simulink model "Cell_v1"  (R2012b)
settings: Solver=ode45  StartTime=0.0  StopTime=1000  RelTol=1e-3
values from neighbouring files (symbols this model uses):
  l_addasrna_rate_1 = g_addasrna_rate    (= 0)    [run_cell.m]
  l_addasrna_rate_2 = g_addasrna_rate    (= 0)    [run_cell.m]
  l_addasrna_rate_3 = 0.01    [run_cell.m]
  l_addasrna_rate_4 = g_addasrna_rate    (= 0)    [run_cell.m]
  l_asrna_die_rate = 0.01    [run_cell.m]
  l_eaten_rate = 0.001    [run_cell.m]
  l_nuk_die_rate = 0.009    [run_cell.m]
  l_pol_die_rate = 0.01    [run_cell.m]
  l_queue_time = 1    [run_cell.m]
  l_rib_die_rate = 0.004    [run_cell.m]
  l_rib_serv_rate = 0.01    [run_cell.m]
  n_asrna = 3    [run_cell.m]
  n_rib = n_initial_rib    (= 15)    [run_cell.m]
  n_rnk_nuk = a    (= 15)    [run_cell.m]
  n_rnk_pol = n_initial_pol    (= 15)    [run_cell.m]
  seed = (seed-321)    (= 12025)    [run_cell.m]
undefined symbols (not defined in the file or in its folder): des, gcbh, PacketRate
libraries: simulink x3
settings Model: Creator=Alex  LastModifiedBy=Alex
settings DataIOCC: InspectSignalLogs=on
settings ConfigurationSet: Description=SimMechanics 2G

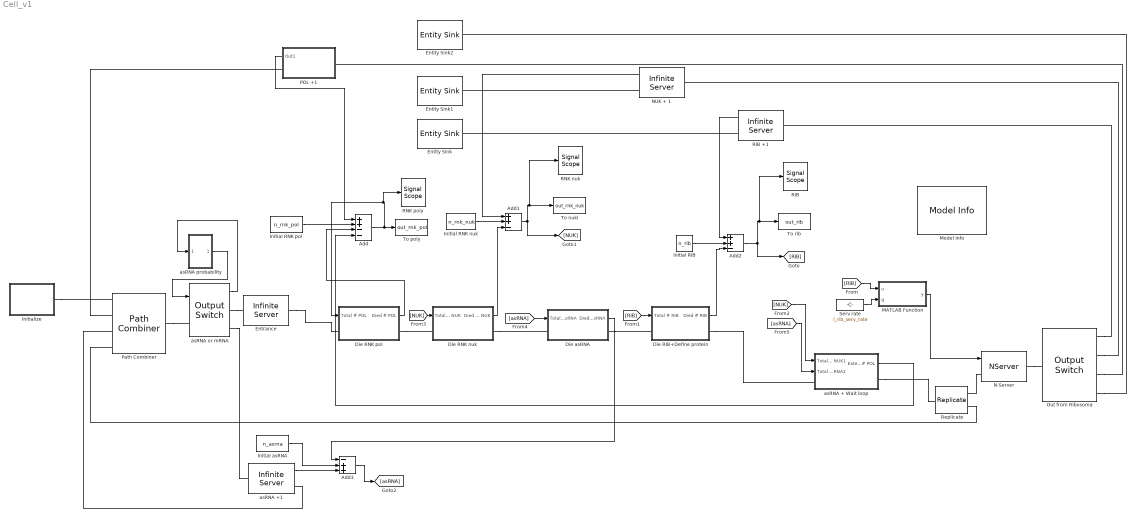
== system Cell_v1 ==
  Add : Sum  Inputs=++--
  Add1 : Sum  Inputs=++-
  Add2 : Sum  Inputs=++-
  Add3 : Sum  Inputs=-++
  Die RIB+Define protein : Subsystem
  Die RNK nuk : Subsystem
  Die RNK pol : Subsystem
  Die asRNA : Subsystem
  Entity Sink : EntitySink
  Entity Sink1 : EntitySink
  Entity Sink2 : EntitySink
  Entrance : InfiniteServer  ServiceTime=0
  Initial RIB : Constant  Value=n_rib
  Initial RNK nuk : Constant  Value=n_rnk_nuk
  Initial RNK pol : Constant  Value=n_rnk_pol
  Initial asRNA : Constant  Value=n_asrna
  Initialize : Subsystem
  MATLAB Function : MATLAB Function  TreatAsAtomicUnit=on
  Model Info : simulink/Model-Wide Utilities/Model Info  InitialBlockCM=None  BlockCM=None  Frame=on  DisplayStringWithTags=|  HorizontalTextAlignment=Center  LeftAlignmentValue=0.5  SourceBlockDiagram=Cell_v1  TagMaxNumber=20
      | Model Info
      | 1 - Ribosome
      | 2 - RNK nuclease
      | 3 - RNK polymerase
  N-Server : NServer  NumberOfServers=n_rib  ServiceTimeFrom=Signal port t  ServiceTime=2
  NUK + 1 : InfiniteServer  ServiceTime=0  StatNumberDeparted=on
  Out from Ribosoma : OutputSwitch  NumberOutputPorts=4  SwitchingCriterion=From attribute  AttributeName=Protein
  POL +1 : Subsystem
  Path Combiner : PathCombiner  NumberInputPorts=4
  RIB : SignalScope  LoadFcn=des.scope.CallbackSupport('seLoadFcn',gcbh)  StartFcn=des.scope.CallbackSupport('seStartFcn',gcbh)  StopFcn=des.scope.CallbackSupport('seStopFcn',gcbh)  XLabel=Time  YLabel=Total Number of Entities  ShowCountPlotted=on  DataStoreOption=Unlimited
      settings: CopyFcn=des.scope.CallbackSupport('seCopyFcn',gcbh)  DeleteFcn=des.scope.CallbackSupport('seDeleteFcn',gcbh)  PreSaveFcn=des.scope.CallbackSupport('sePreSaveFcn',gcbh)  NameChangeFcn=des.scope.CallbackSupport('seNameChangeFcn',gcbh)  OpenFcn=des.scope.CallbackSupport('seOpenFcn',gcbh)
  RIB +1 : InfiniteServer  ServiceTime=0  StatNumberDeparted=on
  RNK nuk : SignalScope  LoadFcn=des.scope.CallbackSupport('seLoadFcn',gcbh)  StartFcn=des.scope.CallbackSupport('seStartFcn',gcbh)  StopFcn=des.scope.CallbackSupport('seStopFcn',gcbh)  XLabel=Time  YLabel=Total Number of Entities  DataStoreOption=Unlimited
      settings: CopyFcn=des.scope.CallbackSupport('seCopyFcn',gcbh)  DeleteFcn=des.scope.CallbackSupport('seDeleteFcn',gcbh)  PreSaveFcn=des.scope.CallbackSupport('sePreSaveFcn',gcbh)  NameChangeFcn=des.scope.CallbackSupport('seNameChangeFcn',gcbh)  OpenFcn=des.scope.CallbackSupport('seOpenFcn',gcbh)
  RNK poly : SignalScope  LoadFcn=des.scope.CallbackSupport('seLoadFcn',gcbh)  StartFcn=des.scope.CallbackSupport('seStartFcn',gcbh)  StopFcn=des.scope.CallbackSupport('seStopFcn',gcbh)  XLabel=Time  YLabel=Total Number of Entities  DataStoreOption=Unlimited
      settings: CopyFcn=des.scope.CallbackSupport('seCopyFcn',gcbh)  DeleteFcn=des.scope.CallbackSupport('seDeleteFcn',gcbh)  PreSaveFcn=des.scope.CallbackSupport('sePreSaveFcn',gcbh)  NameChangeFcn=des.scope.CallbackSupport('seNameChangeFcn',gcbh)  OpenFcn=des.scope.CallbackSupport('seOpenFcn',gcbh)
  Replicate : Replicate  NumberOutputPorts=2
  Serv rate : Constant  Value=l_rib_serv_rate
  To nukl : ToWorkspace  VariableName=out_rnk_nuk  SampleTime=-1  SaveFormat=Timeseries
  To poly : ToWorkspace  VariableName=out_rnk_pol  SampleTime=-1  SaveFormat=Timeseries
  To rib : ToWorkspace  VariableName=out_rib  SampleTime=-1  SaveFormat=Timeseries
  asRNA + Wait loop : Subsystem
  asRNA +1 : InfiniteServer  ServiceTime=0  StatNumberDeparted=on
  asRNA or mRNA : OutputSwitch  NumberOutputPorts=2  SwitchingCriterion=From signal port p  StatNumberDeparted=on
  asRNA probability : Subsystem
  wires:
  Die RNK nuk/1(Died # NUK) -> Add1/3
  Die RIB+Define protein/1(Died # RIB) -> Add2/3
  Die RNK pol/1(Died # POL) -> Add/3
  NUK + 1/1 -> Add1/1
  Add1/1 -> RNK nuk/1, To nukl/1, [NUK]
  RIB +1/1 -> Add2/1
  Add/1 -> To poly/1, RNK poly/1, Die RNK pol/1(Total # POL)
  Initial RNK pol/1 -> Add/2
  Initial RNK nuk/1 -> Add1/2
  Initial RIB/1 -> Add2/2
  MATLAB Function/1(y) -> N-Server/1
  POL +1/1(Out1) -> Add/1
  asRNA + Wait loop/1(Eaten # POL) -> Add/4
  [RIB] -> MATLAB Function/1(u)
  [RIB] -> Die RIB+Define protein/1(Total # RIB)
  Add2/1 -> RIB/1, To rib/1, [RIB]
  [NUK] -> asRNA + Wait loop/1(Total # NUK1)
  [NUK] -> Die RNK nuk/1(Total # NUK)
  Serv rate/1 -> MATLAB Function/2(g)
  asRNA or mRNA/1 -> asRNA probability/1(In1)
  asRNA probability/1(Out1) -> asRNA or mRNA/1
  asRNA +1/1 -> Add3/3
  Initial asRNA/1 -> Add3/2
  [asRNA] -> Die asRNA/1(Total # asRNA)
  Die asRNA/1(Died # asRNA) -> Add3/1
  [asRNA] -> asRNA + Wait loop/2(Total # asRNA2)
  Add3/1 -> [asRNA]
  connections:
  RIB +1/RConn1 -- Entity Sink/LConn1
  Out from Ribosoma/RConn2 -- NUK + 1/LConn1
  NUK + 1/RConn1 -- Entity Sink1/LConn1
  Out from Ribosoma/RConn1 -- RIB +1/LConn1
  Initialize/RConn1 -- Path Combiner/LConn1
  Die RNK pol/RConn1 -- Die RNK nuk/LConn1
  Die asRNA/RConn1 -- Die RIB+Define protein/LConn1
  Entrance/RConn1 -- Die RNK pol/LConn1
  Out from Ribosoma/RConn4 -- Entity Sink2/LConn1
  POL +1/RConn1 -- Path Combiner/LConn2
  Out from Ribosoma/RConn3 -- POL +1/LConn1
  asRNA + Wait loop/RConn1 -- Replicate/LConn1
  N-Server/RConn1 -- Out from Ribosoma/LConn1
  Replicate/RConn1 -- N-Server/LConn1
  Replicate/RConn2 -- Path Combiner/LConn4
  Path Combiner/RConn1 -- asRNA or mRNA/LConn1
  asRNA or mRNA/RConn1 -- Entrance/LConn1
  asRNA or mRNA/RConn2 -- asRNA +1/LConn1
  asRNA +1/RConn1 -- Path Combiner/LConn3
  Die RNK nuk/RConn1 -- Die asRNA/LConn1
  Die RIB+Define protein/RConn1 -- asRNA + Wait loop/LConn1

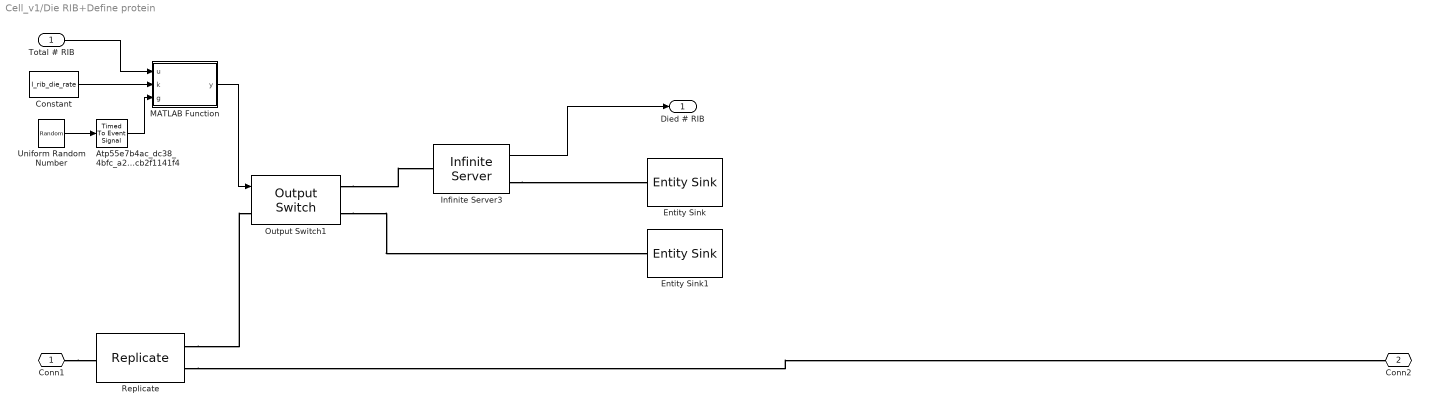
== system Cell_v1/Die RIB+Define protein ==
  Total # RIB : Inport
  Atp55e7b4ac_dc38_4bfc_a2da_90cb2f1141f4 : TimedToEventSignal
  Constant : Constant  Value=l_rib_die_rate
  Entity Sink : EntitySink
  Entity Sink1 : EntitySink
  Infinite Server3 : InfiniteServer  ServiceTime=0  StatNumberDeparted=on
  MATLAB Function : MATLAB Function  TreatAsAtomicUnit=on
  Output Switch1 : OutputSwitch  NumberOutputPorts=2  SwitchingCriterion=From signal port p  InitialConditionsOpt=on  InitialConditions=2
  Replicate : Replicate  NumberOutputPorts=2
  Uniform Random Number : UniformRandomNumber  Minimum=-0.5  Maximum=0.5  Seed=seed  SampleTime=0
  Conn1 : PMIOPort  Port=1  Side=Left
  Conn2 : PMIOPort  Port=2  Side=Right
  Died # RIB : Outport
  wires:
  Infinite Server3/1 -> Died # RIB/1
  MATLAB Function/1(y) -> Output Switch1/1
  Uniform Random Number/1 -> Atp55e7b4ac_dc38_4bfc_a2da_90cb2f1141f4/1
  Atp55e7b4ac_dc38_4bfc_a2da_90cb2f1141f4/1 -> MATLAB Function/3(g)
  Total # RIB/1 -> MATLAB Function/1(u)
  Constant/1 -> MATLAB Function/2(k)
  connections:
  Replicate/RConn1 -- Output Switch1/LConn1
  Infinite Server3/RConn1 -- Entity Sink/LConn1
  Conn1/RConn1 -- Replicate/LConn1
  Output Switch1/RConn1 -- Infinite Server3/LConn1
  Output Switch1/RConn2 -- Entity Sink1/LConn1
  Replicate/RConn2 -- Conn2/RConn1

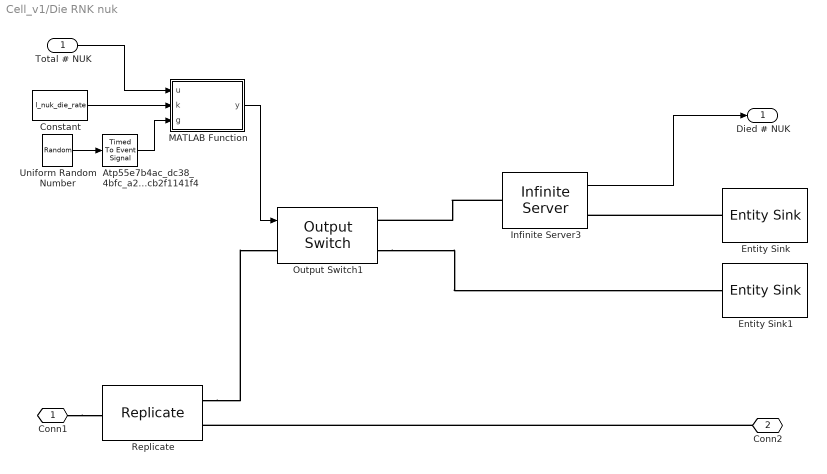
== system Cell_v1/Die RNK nuk ==
  Total # NUK : Inport
  Atp55e7b4ac_dc38_4bfc_a2da_90cb2f1141f4 : TimedToEventSignal
  Constant : Constant  Value=l_nuk_die_rate
  Entity Sink : EntitySink
  Entity Sink1 : EntitySink
  Infinite Server3 : InfiniteServer  ServiceTime=0  StatNumberDeparted=on
  MATLAB Function : MATLAB Function  TreatAsAtomicUnit=on
  Output Switch1 : OutputSwitch  NumberOutputPorts=2  SwitchingCriterion=From signal port p  InitialConditionsOpt=on  InitialConditions=2
  Replicate : Replicate  NumberOutputPorts=2
  Uniform Random Number : UniformRandomNumber  Minimum=-0.5  Maximum=0.5  Seed=seed  SampleTime=0
  Conn1 : PMIOPort  Port=1  Side=Left
  Conn2 : PMIOPort  Port=2  Side=Right
  Died # NUK : Outport
  wires:
  Infinite Server3/1 -> Died # NUK/1
  MATLAB Function/1(y) -> Output Switch1/1
  Uniform Random Number/1 -> Atp55e7b4ac_dc38_4bfc_a2da_90cb2f1141f4/1
  Atp55e7b4ac_dc38_4bfc_a2da_90cb2f1141f4/1 -> MATLAB Function/3(g)
  Total # NUK/1 -> MATLAB Function/1(u)
  Constant/1 -> MATLAB Function/2(k)
  connections:
  Entity Sink/LConn1 -- Infinite Server3/RConn1
  Replicate/RConn1 -- Output Switch1/LConn1
  Conn1/RConn1 -- Replicate/LConn1
  Conn2/RConn1 -- Replicate/RConn2
  Infinite Server3/LConn1 -- Output Switch1/RConn1
  Output Switch1/RConn2 -- Entity Sink1/LConn1

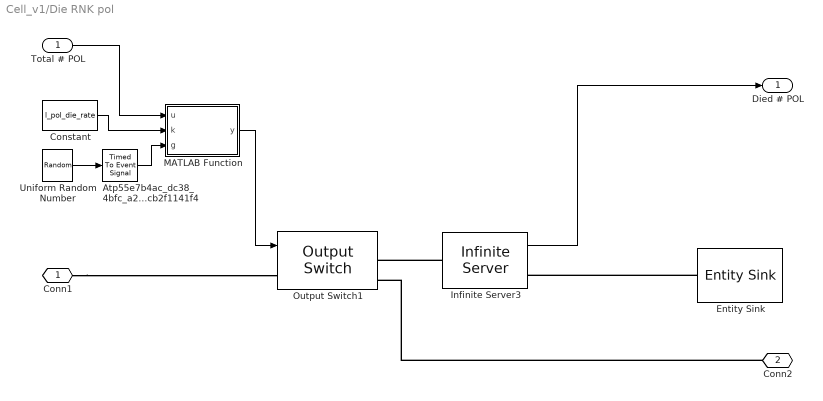
== system Cell_v1/Die RNK pol ==
  Total # POL : Inport
  Atp55e7b4ac_dc38_4bfc_a2da_90cb2f1141f4 : TimedToEventSignal
  Constant : Constant  Value=l_pol_die_rate
  Entity Sink : EntitySink
  Infinite Server3 : InfiniteServer  ServiceTime=0  StatNumberDeparted=on
  MATLAB Function : MATLAB Function  TreatAsAtomicUnit=on
  Output Switch1 : OutputSwitch  NumberOutputPorts=2  SwitchingCriterion=From signal port p  InitialConditionsOpt=on  InitialConditions=2  StatLastDeparturePort=on
      settings: OutputPortMap=o3
  Uniform Random Number : UniformRandomNumber  Minimum=-0.5  Maximum=0.5  Seed=seed  SampleTime=0
  Conn1 : PMIOPort  Port=1  Side=Left
  Conn2 : PMIOPort  Port=2  Side=Right
  Died # POL : Outport
  wires:
  Infinite Server3/1 -> Died # POL/1
  Uniform Random Number/1 -> Atp55e7b4ac_dc38_4bfc_a2da_90cb2f1141f4/1
  Atp55e7b4ac_dc38_4bfc_a2da_90cb2f1141f4/1 -> MATLAB Function/3(g)
  Total # POL/1 -> MATLAB Function/1(u)
  MATLAB Function/1(y) -> Output Switch1/1
  Constant/1 -> MATLAB Function/2(k)
  connections:
  Entity Sink/LConn1 -- Infinite Server3/RConn1
  Infinite Server3/LConn1 -- Output Switch1/RConn1
  Conn2/RConn1 -- Output Switch1/RConn2
  Conn1/RConn1 -- Output Switch1/LConn1

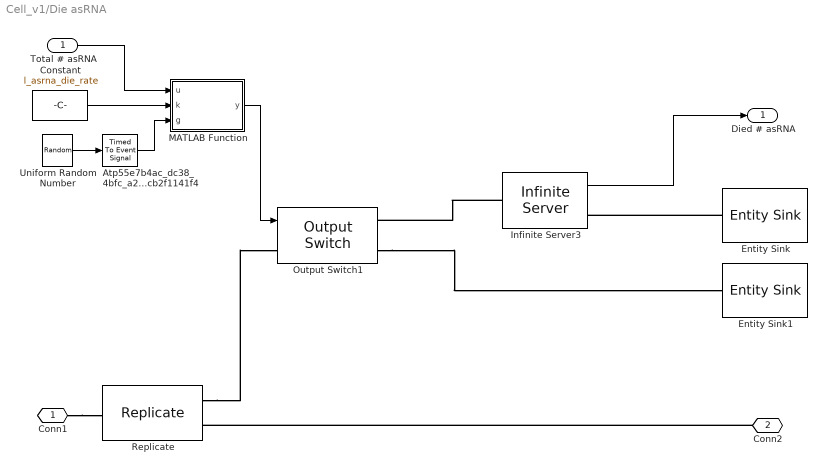
== system Cell_v1/Die asRNA ==
  Total # asRNA : Inport
  Atp55e7b4ac_dc38_4bfc_a2da_90cb2f1141f4 : TimedToEventSignal
  Constant : Constant  Value=l_asrna_die_rate
  Entity Sink : EntitySink
  Entity Sink1 : EntitySink
  Infinite Server3 : InfiniteServer  ServiceTime=0  StatNumberDeparted=on
  MATLAB Function : MATLAB Function  TreatAsAtomicUnit=on
  Output Switch1 : OutputSwitch  NumberOutputPorts=2  SwitchingCriterion=From signal port p  InitialConditionsOpt=on  InitialConditions=2
  Replicate : Replicate  NumberOutputPorts=2
  Uniform Random Number : UniformRandomNumber  Minimum=-0.5  Maximum=0.5  Seed=seed  SampleTime=0
  Conn1 : PMIOPort  Port=1  Side=Left
  Conn2 : PMIOPort  Port=2  Side=Right
  Died # asRNA : Outport
  wires:
  Infinite Server3/1 -> Died # asRNA/1
  MATLAB Function/1(y) -> Output Switch1/1
  Uniform Random Number/1 -> Atp55e7b4ac_dc38_4bfc_a2da_90cb2f1141f4/1
  Atp55e7b4ac_dc38_4bfc_a2da_90cb2f1141f4/1 -> MATLAB Function/3(g)
  Total # asRNA/1 -> MATLAB Function/1(u)
  Constant/1 -> MATLAB Function/2(k)
  connections:
  Entity Sink/LConn1 -- Infinite Server3/RConn1
  Replicate/RConn1 -- Output Switch1/LConn1
  Conn1/RConn1 -- Replicate/LConn1
  Conn2/RConn1 -- Replicate/RConn2
  Infinite Server3/LConn1 -- Output Switch1/RConn1
  Output Switch1/RConn2 -- Entity Sink1/LConn1

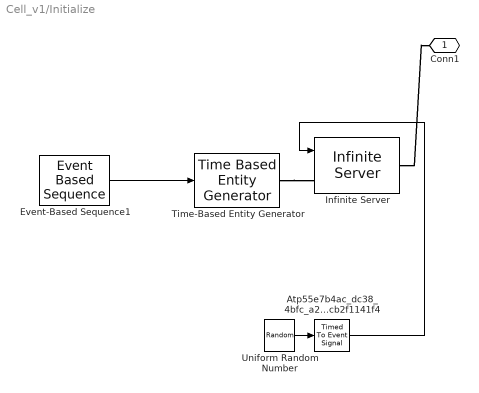
== system Cell_v1/Initialize ==
  Atp55e7b4ac_dc38_4bfc_a2da_90cb2f1141f4 : TimedToEventSignal
  Event-Based Sequence1 : EventBasedSequence  VectorOutputValues=p_initial_pol  FormOutputOpt=Setting to infinity
  Infinite Server : InfiniteServer  ServiceTimeFrom=Signal port t
  Time-Based Entity Generator : TimeBasedEntityGenerator  GenerateEntitiesUpon=Intergeneration time from port t  Distribution=Uniform
  Uniform Random Number : UniformRandomNumber  Minimum=0  Seed=seed  SampleTime=0
  Conn1 : PMIOPort  Port=1  Side=Right
  wires:
  Uniform Random Number/1 -> Atp55e7b4ac_dc38_4bfc_a2da_90cb2f1141f4/1
  Event-Based Sequence1/1 -> Time-Based Entity Generator/1
  Atp55e7b4ac_dc38_4bfc_a2da_90cb2f1141f4/1 -> Infinite Server/1
  connections:
  Time-Based Entity Generator/RConn1 -- Infinite Server/LConn1
  Infinite Server/RConn1 -- Conn1/RConn1

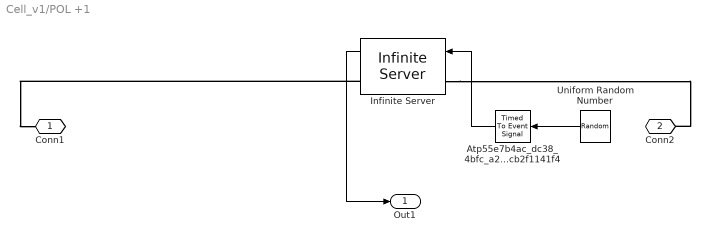
== system Cell_v1/POL +1 ==
  Atp55e7b4ac_dc38_4bfc_a2da_90cb2f1141f4 : TimedToEventSignal
  Infinite Server : InfiniteServer  ServiceTimeFrom=Signal port t  ServiceTime=0  StatNumberDeparted=on
  Uniform Random Number : UniformRandomNumber  Minimum=0  Seed=seed  SampleTime=0
  Conn1 : PMIOPort  Port=1  Side=Right
  Conn2 : PMIOPort  Port=2  Side=Left
  Out1 : Outport
  wires:
  Infinite Server/1 -> Out1/1
  Uniform Random Number/1 -> Atp55e7b4ac_dc38_4bfc_a2da_90cb2f1141f4/1
  Atp55e7b4ac_dc38_4bfc_a2da_90cb2f1141f4/1 -> Infinite Server/1
  connections:
  Infinite Server/LConn1 -- Conn2/RConn1
  Infinite Server/RConn1 -- Conn1/RConn1

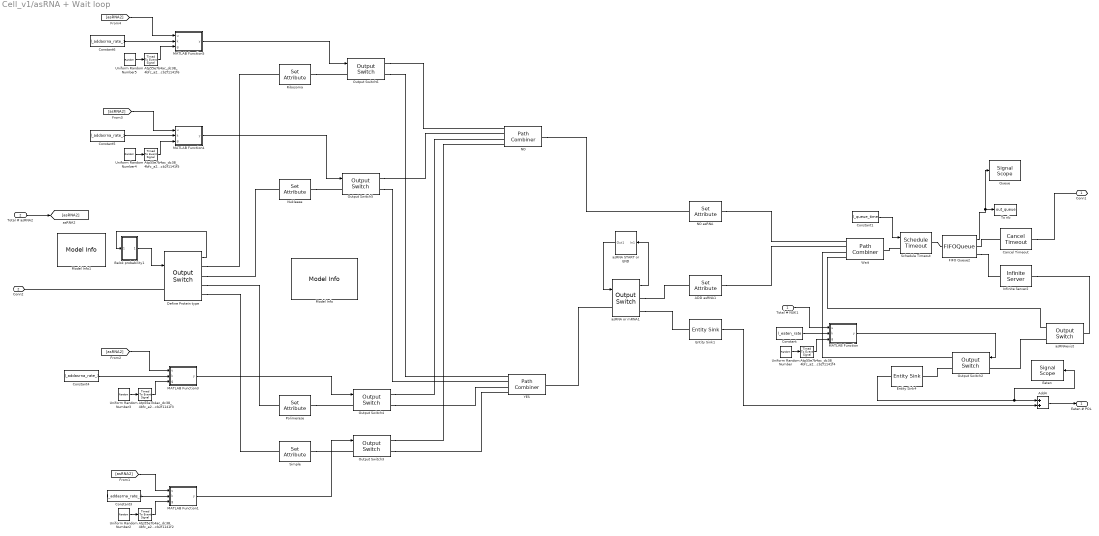
== system Cell_v1/asRNA + Wait loop ==
  Total # NUK1 : Inport
  Total # asRNA2 : Inport  Port=2
  ADD asRNA1 : SetAttribute  AttributeName=asRNAexist  EvaluatedAttributeValue={ 1 }
  Add4 : Sum
  Atp55e7b4ac_dc38_4bfc_a2da_90cb2f1141f{2..6} (5 alike) : TimedToEventSignal
  Belok probability1 : Subsystem
  Cancel Timeout : CancelTimeout
  Constant : Constant  Value=l_eaten_rate
  Constant1 : Constant  Value=l_queue_time
  Constant3 : Constant  Value=l_addasrna_rate_4
  Constant4 : Constant  Value=l_addasrna_rate_3
  Constant5 : Constant  Value=l_addasrna_rate_2
  Constant6 : Constant  Value=l_addasrna_rate_1
  Define Protein type : OutputSwitch  NumberOutputPorts=4  SwitchingCriterion=From signal port p  StatNumberDeparted=on
  Eaten : SignalScope  LoadFcn=des.scope.CallbackSupport('seLoadFcn',gcbh)  StartFcn=des.scope.CallbackSupport('seStartFcn',gcbh)  StopFcn=des.scope.CallbackSupport('seStopFcn',gcbh)
      settings: CopyFcn=des.scope.CallbackSupport('seCopyFcn',gcbh)  DeleteFcn=des.scope.CallbackSupport('seDeleteFcn',gcbh)  PreSaveFcn=des.scope.CallbackSupport('sePreSaveFcn',gcbh)  NameChangeFcn=des.scope.CallbackSupport('seNameChangeFcn',gcbh)  OpenFcn=des.scope.CallbackSupport('seOpenFcn',gcbh)
  Entity Sink1 : EntitySink  StatNumberArrived=on
  Entity Sink4 : EntitySink  StatNumberArrived=on
  FIFO Queue2 : FIFOQueue  Capacity=10000  EnableTOPort=on  StatAverageQueueLength=on
      settings: OutputPortMap=o3
  Infinite Server2 : InfiniteServer  ServiceTime=0
  MATLAB Function : MATLAB Function  TreatAsAtomicUnit=on
  MATLAB Function1 : MATLAB Function  TreatAsAtomicUnit=on
  MATLAB Function3 : MATLAB Function  TreatAsAtomicUnit=on
  MATLAB Function4 : MATLAB Function  TreatAsAtomicUnit=on
  MATLAB Function5 : MATLAB Function  TreatAsAtomicUnit=on
  Model Info : simulink/Model-Wide Utilities/Model Info  InitialBlockCM=None  BlockCM=None  Frame=on  DisplayStringWithTags=|  HorizontalTextAlignment=Center  LeftAlignmentValue=0.5  SourceBlockDiagram=Cell_v1  TagMaxNumber=20
      | Add asRNA
      | 1 - NO, asRNA was NOT added
      | 2 - YES, asRNA was added
  Model Info1 : simulink/Model-Wide Utilities/Model Info  InitialBlockCM=None  BlockCM=None  Frame=on  DisplayStringWithTags=|  HorizontalTextAlignment=Center  LeftAlignmentValue=0.5  SourceBlockDiagram=Cell_v1  TagMaxNumber=20
      | Model Info
      | 1 - Ribosome
      | 2 - RNK nuclease
      | 3 - RNK polymerase
  NO : PathCombiner  NumberInputPorts=4
  NO asRNA : SetAttribute  AttributeName=asRNAexist  AttributeValue=2  EvaluatedAttributeValue={ 2 }
  Nuklease : SetAttribute  AttributeName=Protein  AttributeValue=2  EvaluatedAttributeValue={ 2 }
  Output Switch2 : OutputSwitch  NumberOutputPorts=2  SwitchingCriterion=From signal port p  InitialConditionsOpt=on
  Output Switch{3..6} (4 alike) : OutputSwitch  NumberOutputPorts=2  SwitchingCriterion=From signal port p
  Polimerase : SetAttribute  AttributeName=Protein  AttributeValue=3  EvaluatedAttributeValue={ 3 }
  Queue : SignalScope  LoadFcn=des.scope.CallbackSupport('seLoadFcn',gcbh)  StartFcn=des.scope.CallbackSupport('seStartFcn',gcbh)  StopFcn=des.scope.CallbackSupport('seStopFcn',gcbh)
      settings: CopyFcn=des.scope.CallbackSupport('seCopyFcn',gcbh)  DeleteFcn=des.scope.CallbackSupport('seDeleteFcn',gcbh)  PreSaveFcn=des.scope.CallbackSupport('sePreSaveFcn',gcbh)  NameChangeFcn=des.scope.CallbackSupport('seNameChangeFcn',gcbh)  OpenFcn=des.scope.CallbackSupport('seOpenFcn',gcbh)
  Ribosoma : SetAttribute  AttributeName=Protein  EvaluatedAttributeValue={ 1 }
  Schedule Timeout : ScheduleTimeout  TimeoutIntervalFrom=Signal port ti  TimeoutInterval=2
  Simple : SetAttribute  AttributeName=Protein  AttributeValue=4  EvaluatedAttributeValue={ 4 }
  To rib : ToWorkspace  VariableName=out_queue  SampleTime=-1  SaveFormat=Timeseries
  Uniform Random Number{,2..5} (5 alike) : UniformRandomNumber  Minimum=-0.5  Maximum=0.5  Seed=seed  SampleTime=0
  Wait : PathCombiner  NumberInputPorts=4
  YES : PathCombiner  NumberInputPorts=4
  asRNA START or END : Subsystem
  asRNA or mRNA1 : OutputSwitch  NumberOutputPorts=2  SwitchingCriterion=From signal port p  StatNumberDeparted=on
  asRNAexist : OutputSwitch  NumberOutputPorts=2  SwitchingCriterion=From attribute  AttributeName=asRNAexist  InitialConditionsOpt=on
  Conn1 : PMIOPort  Port=1  Side=Right
  Conn2 : PMIOPort  Port=2  Side=Left
  Eaten # POL : Outport
  wires:
  Entity Sink4/1 -> Eaten/1, Add4/1
  Uniform Random Number/1 -> Atp55e7b4ac_dc38_4bfc_a2da_90cb2f1141f4/1
  Atp55e7b4ac_dc38_4bfc_a2da_90cb2f1141f4/1 -> MATLAB Function/3(g)
  Total # NUK1/1 -> MATLAB Function/1(u)
  MATLAB Function/1(y) -> Output Switch2/1
  Constant/1 -> MATLAB Function/2(k)
  Constant1/1 -> Schedule Timeout/1
  asRNA or mRNA1/1 -> asRNA START or END/1(In1)
  asRNA START or END/1(Out1) -> asRNA or mRNA1/1
  Entity Sink1/1 -> Add4/2
  Add4/1 -> Eaten # POL/1
  Define Protein type/1 -> Belok probability1/1(In1)
  Belok probability1/1(Out1) -> Define Protein type/1
  Uniform Random Number2/1 -> Atp55e7b4ac_dc38_4bfc_a2da_90cb2f1141f2/1
  Atp55e7b4ac_dc38_4bfc_a2da_90cb2f1141f2/1 -> MATLAB Function1/3(g)
  Constant3/1 -> MATLAB Function1/2(k)
  MATLAB Function1/1(y) -> Output Switch3/1
  Uniform Random Number3/1 -> Atp55e7b4ac_dc38_4bfc_a2da_90cb2f1141f3/1
  Atp55e7b4ac_dc38_4bfc_a2da_90cb2f1141f3/1 -> MATLAB Function3/3(g)
  Constant4/1 -> MATLAB Function3/2(k)
  MATLAB Function3/1(y) -> Output Switch4/1
  Uniform Random Number4/1 -> Atp55e7b4ac_dc38_4bfc_a2da_90cb2f1141f5/1
  Atp55e7b4ac_dc38_4bfc_a2da_90cb2f1141f5/1 -> MATLAB Function4/3(g)
  [asRNA2] -> MATLAB Function4/1(u)
  Constant5/1 -> MATLAB Function4/2(k)
  MATLAB Function4/1(y) -> Output Switch5/1
  Uniform Random Number5/1 -> Atp55e7b4ac_dc38_4bfc_a2da_90cb2f1141f6/1
  Atp55e7b4ac_dc38_4bfc_a2da_90cb2f1141f6/1 -> MATLAB Function5/3(g)
  [asRNA2] -> MATLAB Function5/1(u)
  Constant6/1 -> MATLAB Function5/2(k)
  MATLAB Function5/1(y) -> Output Switch6/1
  Total # asRNA2/1 -> [asRNA2]
  [asRNA2] -> MATLAB Function3/1(u)
  [asRNA2] -> MATLAB Function1/1(u)
  FIFO Queue2/1 -> Queue/1, To rib/1
  connections:
  FIFO Queue2/RConn2 -- Infinite Server2/LConn1
  Wait/LConn3 -- Output Switch2/RConn1
  Wait/RConn1 -- Schedule Timeout/LConn1
  Output Switch2/RConn2 -- Entity Sink4/LConn1
  Cancel Timeout/RConn1 -- Conn1/RConn1
  Schedule Timeout/RConn1 -- FIFO Queue2/LConn1
  FIFO Queue2/RConn1 -- Cancel Timeout/LConn1
  Infinite Server2/RConn1 -- asRNAexist/LConn1
  asRNAexist/RConn1 -- Wait/LConn4
  asRNAexist/RConn2 -- Output Switch2/LConn1
  asRNA or mRNA1/LConn1 -- YES/RConn1
  asRNA or mRNA1/RConn1 -- ADD asRNA1/LConn1
  asRNA or mRNA1/RConn2 -- Entity Sink1/LConn1
  NO/RConn1 -- NO asRNA/LConn1
  NO asRNA/RConn1 -- Wait/LConn1
  ADD asRNA1/RConn1 -- Wait/LConn2
  Define Protein type/RConn2 -- Nuklease/LConn1
  Define Protein type/LConn1 -- Conn2/RConn1
  Ribosoma/RConn1 -- Output Switch6/LConn1
  Nuklease/RConn1 -- Output Switch5/LConn1
  Simple/RConn1 -- Output Switch3/LConn1
  Define Protein type/RConn3 -- Polimerase/LConn1
  Define Protein type/RConn1 -- Ribosoma/LConn1
  Define Protein type/RConn4 -- Simple/LConn1
  Polimerase/RConn1 -- Output Switch4/LConn1
  Output Switch6/RConn1 -- NO/LConn1
  Output Switch5/RConn1 -- NO/LConn2
  Output Switch4/RConn1 -- NO/LConn3
  Output Switch3/RConn1 -- NO/LConn4
  Output Switch4/RConn2 -- YES/LConn3
  Output Switch3/RConn2 -- YES/LConn4
  Output Switch6/RConn2 -- YES/LConn1
  Output Switch5/RConn2 -- YES/LConn2

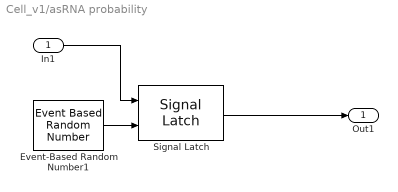
== system Cell_v1/asRNA probability ==
  In1 : Inport
  Event-Based Random Number1 : EventBasedRandomNumber  Distribution=Arbitrary discrete  meanExp=1/PacketRate  minUnif=1  maxUnif=MaxPacketSize  valueVecDisc=[1 2]  probVecDisc=p_RNA_routing  Seed=seed
  Signal Latch : SignalLatch  InitialMemoryValue=2  ReadMemoryUpon=Write to memory event
      settings: InputPortMap=u0,u2  OutputPortMap=o2
  Out1 : Outport
  wires:
  Event-Based Random Number1/1 -> Signal Latch/2
  Signal Latch/1 -> Out1/1
  In1/1 -> Signal Latch/1

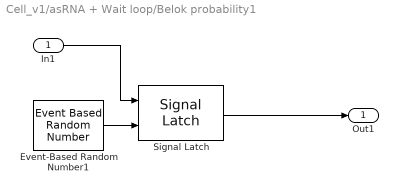
== system Cell_v1/asRNA + Wait loop/Belok probability1 ==
  In1 : Inport
  Event-Based Random Number1 : EventBasedRandomNumber  Distribution=Arbitrary discrete  meanExp=1/PacketRate  minUnif=1  maxUnif=MaxPacketSize  valueVecDisc=[1 2 3 4]  probVecDisc=p_routing  Seed=seed
  Signal Latch : SignalLatch  InitialMemoryValue=2  ReadMemoryUpon=Write to memory event
      settings: InputPortMap=u0,u2  OutputPortMap=o2
  Out1 : Outport
  wires:
  Event-Based Random Number1/1 -> Signal Latch/2
  Signal Latch/1 -> Out1/1
  In1/1 -> Signal Latch/1

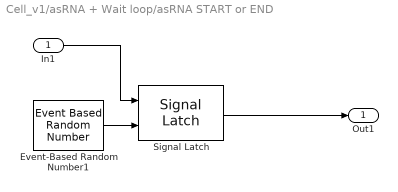
== system Cell_v1/asRNA + Wait loop/asRNA START or END ==
  In1 : Inport
  Event-Based Random Number1 : EventBasedRandomNumber  Distribution=Arbitrary discrete  meanExp=1/PacketRate  minUnif=1  maxUnif=MaxPacketSize  valueVecDisc=[1 2]  probVecDisc=p_asRNA_start_end  Seed=seed
  Signal Latch : SignalLatch  InitialMemoryValue=2  ReadMemoryUpon=Write to memory event
      settings: InputPortMap=u0,u2  OutputPortMap=o2
  Out1 : Outport
  wires:
  Event-Based Random Number1/1 -> Signal Latch/2
  Signal Latch/1 -> Out1/1
  In1/1 -> Signal Latch/1

== matlab function Cell_v1/Die RIB+Define protein/MATLAB Function ==
  data: u input; k input; y output; g input
function y = fcnRIB(u,k,g)
y =1+round(g + exp(-k*u));

== matlab function Cell_v1/MATLAB Function ==
  data: u input; y output; g input
function y = TimeInServer(u,g)
%#codegen
k = rand(1);

y = 10*exp(-g*u)*(1+0.2*(k-0.5));

== matlab function Cell_v1/Die RNK nuk/MATLAB Function ==
  data: u input; k input; y output; g input
function y = fcnNUK(u,k,g)
y =1+round(g + exp(-k*u));

== matlab function Cell_v1/asRNA + Wait loop/MATLAB Function ==
  data: u input; k input; y output; g input
function y = fcnPOL(u,k,g)
y =1+round(g + 1-exp(-k*u));

== matlab function Cell_v1/Die asRNA/MATLAB Function ==
  data: u input; k input; y output; g input
function y = fcnNUK(u,k,g)
y =1+round(g + exp(-k*u));

== matlab function Cell_v1/Die RNK pol/MATLAB Function ==
  data: u input; k input; y output; g input
function y = fcnPOL(u,k,g)
y =1+min(round(g + exp(-k*u)+0.1),1) ;

== matlab function Cell_v1/asRNA + Wait loop/MATLAB Function1 ==
  data: u input; k input; y output; g input
function y = fcnPOL(u,k,g)
y =1+round(g + 1-exp(-k*u));

== matlab function Cell_v1/asRNA + Wait loop/MATLAB Function3 ==
  data: u input; k input; y output; g input
function y = fcnPOL(u,k,g)
y =1+round(g + 1-exp(-k*u));

== matlab function Cell_v1/asRNA + Wait loop/MATLAB Function4 ==
  data: u input; k input; y output; g input
function y = fcnPOL(u,k,g)
y =1+round(g + 1-exp(-k*u));

== matlab function Cell_v1/asRNA + Wait loop/MATLAB Function5 ==
  data: u input; k input; y output; g input
function y = fcnPOL(u,k,g)
y =1+round(g + 1-exp(-k*u));
